simulink model "NDI_and_CA_Model"  (R2012b)
settings: Solver=FixedStepDiscrete  StartTime=0.0  StopTime=inf  FixedStep=T_sim  MaxStep=0.01  RelTol=1e-5
values from neighbouring files (symbols this model uses):
  A_x = 0.015    [SetupComplete.m]
  A_y = A_x    (= 0.015)    [SetupComplete.m]
  A_z = 0.16    [SetupComplete.m]
  C_x = 1.2    [SetupComplete.m]
  C_y = C_x    (= 1.2)    [SetupComplete.m]
  C_z = 2.2    [SetupComplete.m]
  CG_0 = [0,0,0.02]'    [SetupComplete.m]
  eta_23 = deg2rad(-1.42)    [Run3Copter.m]
  g = 9.81    [SetupComplete.m]
  h_M = 0.064    [SetupComplete.m]
  I_BAC_0 = [ Ix,0,Ixz;0,Iy,0;Ixz,0,Iz]    [SetupComplete.m]
  l = 0.345    [SetupComplete.m]
  l_arm = 0.264    [SetupComplete.m]
  m = 3.51    [SetupComplete.m]
  m_0 = 2.61    [SetupComplete.m]
  m_M = 0.300    (= 0.3)    [SetupComplete.m]
  rho = 1.15    [SetupComplete.m]
  Rotation_sign = [ 1,-1,-1]    [SetupComplete.m]
  throtle_1 = 0.512    [Run3Copter.m]
  throtle_23 = throtle_1/cos(eta_23)    [Run3Copter.m]
  Throttle_Hover = X(1)/16    [SetupComplete.m]
libraries: XXCopter_C x24, simulink_extras x21, aerolibutil x3
(part 1 of 2)
settings Model: ExtModeTrigDuration=5000  Creator=DavidTorres  LastModifiedBy=david.torres
settings SolverCC: SolverResetMethod=Robust  PositivePriorityOrder=on
settings DataIOCC: ExternalInput=getinputstruct(op_trim1)  InitialState=getstatestruct(op_trim1)  SignalLoggingSaveFormat=ModelDataLogs  Refine=10
settings OptimizationCC: InlineParams=on  UseFloatMulNetSlope=on  UseSpecifiedMinMax=on  InlineInvariantSignals=on  EnhancedBackFolding=on  PassReuseOutputArgsAs=Individual arguments  RollThreshold=50  ZeroExternalMemoryAtStartup=off  ZeroInternalMemoryAtStartup=off  EfficientMapNaN2IntZero=off  OptimizeModelRefInitCode=on  LifeSpan=1  MaxStackSize=inf  SimCompilerOptimization=On
settings DebuggingCC: SignalInfNanChecking=warning  WriteAfterReadMsg=DisableAll  UnderspecifiedInitializationDetection=Simplified  MergeDetectMultiDrivingBlocksExec=error  CheckMatrixSingularityMsg=warning  IntegerOverflowMsg=error  Int32ToFloatConvMsg=none  ParameterUnderflowMsg=error  ParameterTunabilityLossMsg=error  UnderSpecifiedDataTypeMsg=warning  UniqueDataStoreMsg=error  AssertControl=DisableAll  ModelReferenceIOMsg=error  StrictBusMsg=ErrorOnBusTreatedAsVector  NonBusSignalsTreatedAsBus=error
settings HardwareCC: ProdIntDivRoundTo=Zero  ProdEndianess=LittleEndian  ProdHWDeviceType=Generic->32-bit x86 compatible  TargetBitPerLong=64  TargetBitPerPointer=64  TargetLargestAtomicInteger=Integer  TargetLargestAtomicFloat=Double  TargetIntDivRoundTo=Zero  TargetEndianess=LittleEndian  TargetWordSize=64  TargetHWDeviceType=Intel->x86-64  ProdEqTarget=off
settings RTWCC: SystemTargetFile=ert.tlc  GenCodeOnly=on  TemplateMakefile=RTW.MSVCBuild  Description=Create Visual C/C++ Solution File for the Embedded Coder  GenerateReport=on  ProcessScript=ert_make_rtw_hook  IncludeHyperlinkInReport=on  LaunchReport=on  CodeExecutionProfiling=on  GenerateTraceInfo=on  RTWCompilerOptimization=On  CheckMdlBeforeBuild=Warning
settings CodeAppCC: IgnoreCustomStorageClasses=off  IgnoreTestpoints=on  MATLABSourceComments=on
settings ERTTargetCC: CodeReplacementLibrary=C89/C90 (ANSI)  UtilityFuncGeneration=Shared location  MultiwordLength=2048  GenerateSampleERTMain=on  IncludeMdlTerminateFcn=off  CombineSignalStateStructs=on  SuppressErrorStatus=on  IncludeFileDelimiter=UseQuote  SupportAbsoluteTime=off  MultiInstanceERTCode=on  SupportComplex=off  ParenthesesLevel=Maximum  InlinedParameterPlacement=NonHierarchical  ERTCustomFileTemplate=example_file_process.tlc  GlobalDataDefinition=InSourceFile  DataDefinitionFile=global_vars.c  GlobalDataReference=InSourceFile  PreserveIfCondition=on  SuppressUnreachableDefaultCases=off

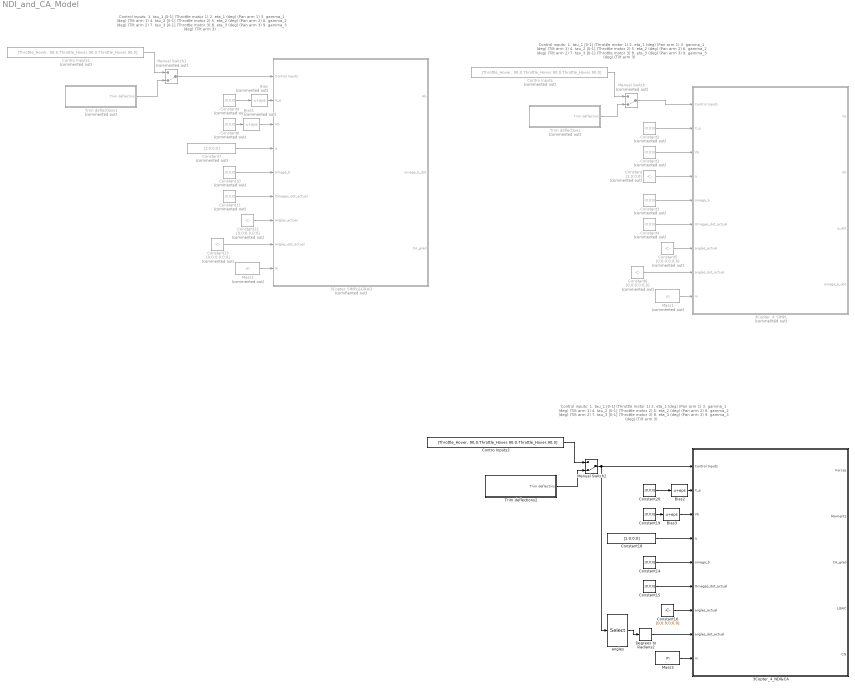
== system NDI_and_CA_Model ==
  note: Control inputs:
      | 1. tau_1 [0-1] (Throttle motor 1)
      | 2. eta_1 (deg)  (Pan arm 1)
      | 3. gamma_1 (deg)  (Tilt arm 1)
      |
      | 4. tau_2 [0-1] (Throttle motor 2)
      | 5. eta_2 (deg)  (Pan arm 2)
      | 6. gamma_2 (deg)  (Tilt arm 2)
      |
      | 7. tau_3 [0-1] (Throttle motor 3)
      | 8. eta_3 (deg)  (Pan arm  3)
      | 9. gamma_3 (deg)  (Tilt arm 3)
  note: Control inputs:
      | 1. tau_1 [0-1] (Throttle motor 1)
      | 2. eta_1 (deg)  (Pan arm 1)
      | 3. gamma_1 (deg)  (Tilt arm 1)
      |
      | 4. tau_2 [0-1] (Throttle motor 2)
      | 5. eta_2 (deg)  (Pan arm 2)
      | 6. gamma_2 (deg)  (Tilt arm 2)
      |
      | 7. tau_3 [0-1] (Throttle motor 3)
      | 8. eta_3 (deg)  (Pan arm  3)
      | 9. gamma_3 (deg)  (Tilt arm 3)
  note: Control inputs:
      | 1. tau_1 [0-1] (Throttle motor 1)
      | 2. eta_1 (deg)  (Pan arm 1)
      | 3. gamma_1 (deg)  (Tilt arm 1)
      |
      | 4. tau_2 [0-1] (Throttle motor 2)
      | 5. eta_2 (deg)  (Pan arm 2)
      | 6. gamma_2 (deg)  (Tilt arm 2)
      |
      | 7. tau_3 [0-1] (Throttle motor 3)
      | 8. eta_3 (deg)  (Pan arm  3)
      | 9. gamma_3 (deg)  (Tilt arm 3)
  3Copter_4_NDI&CA : Subsystem  TreatAsAtomicUnit=on
  3Copter_4_SIMPL : Subsystem  Commented=on  TreatAsAtomicUnit=on
  3Copter_SIMPL&GRAD : Subsystem  Commented=on  TreatAsAtomicUnit=on
  Bias : Bias  Commented=on  Bias=eps
  Bias1 : Bias  Commented=on  Bias=eps
  Bias2 : Bias  Bias=eps
  Bias3 : Bias  Bias=eps
  Constant : Constant  Commented=on  Value=[1;0;0;0]
  Constant{1..4,8..11} (8 alike) : Constant  Commented=on  Value=[0;0;0]
  Constant{5..6,12..13} (4 alike) : Constant  Commented=on  Value=[0;0;0;0;0;0]
  Constant{14..15,19..20} (4 alike) : Constant  Value=[0;0;0]
  Constant16 : Constant  Value=[0;0;0;0;0;0]
  Constant18 : Constant  Value=[1;0;0;0]
  Constant7 : Constant  Commented=on  Value=[1;0;0;0]
  Contro Inputs : Constant  Commented=on  Value=[Throttle_Hover, 90,0,Throttle_Hover,90,0,Throttle_Hover,90,0]
  Contro Inputs1 : Constant  Commented=on  Value=[Throttle_Hover, 90,0,Throttle_Hover,90,0,Throttle_Hover,90,0]
  Contro Inputs2 : Constant  Value=[Throttle_Hover, 90,0,Throttle_Hover,90,0,Throttle_Hover,90,0]
  Degrees to Radians2 : simulink_extras/Transformations/Degrees to Radians
  Manual Switch : ManualSwitch  Commented=on  CurrentSetting=0
  Manual Switch1 : ManualSwitch  Commented=on  CurrentSetting=0
  Manual Switch2 : ManualSwitch  CurrentSetting=0
  Mass1 : Constant  Commented=on  Value=m
  Mass2 : Constant  Commented=on  Value=m
  Mass3 : Constant  Value=m
  Trim deflections : Subsystem  Commented=on  TreatAsAtomicUnit=on
  Trim deflections1 : Subsystem  Commented=on  TreatAsAtomicUnit=on
  Trim deflections2 : Subsystem  TreatAsAtomicUnit=on
  "angles " : Selector  IndexMode=Zero-based  InputPortWidth=9  Indices=[1,2,4,5,7,8]
  wires:
  Manual Switch/1 -> 3Copter_4_SIMPL/1(Control Inputs)
  Contro Inputs/1 -> Manual Switch/1
  Trim deflections/1(Trim deflectins) -> Manual Switch/2
  Constant/1 -> 3Copter_4_SIMPL/4(q)
  Constant1/1 -> 3Copter_4_SIMPL/3(Vb)
  Constant2/1 -> 3Copter_4_SIMPL/2(X_e)
  Constant3/1 -> 3Copter_4_SIMPL/5(omega_b)
  Constant4/1 -> 3Copter_4_SIMPL/6(Omegas_dot_actual)
  Constant5/1 -> 3Copter_4_SIMPL/7(angles_actual)
  Constant6/1 -> 3Copter_4_SIMPL/8(angles_dot_actual)
  Mass1/1 -> 3Copter_4_SIMPL/9(" m")
  Manual Switch1/1 -> 3Copter_SIMPL&GRAD/1(Control Inputs)
  Contro Inputs1/1 -> Manual Switch1/1
  Trim deflections1/1(Trim deflectins) -> Manual Switch1/2
  Constant7/1 -> 3Copter_SIMPL&GRAD/4(q)
  Constant8/1 -> Bias1/1
  Constant9/1 -> Bias/1
  Constant10/1 -> 3Copter_SIMPL&GRAD/5(omega_b)
  Constant11/1 -> 3Copter_SIMPL&GRAD/6(Omegas_dot_actual)
  Constant12/1 -> 3Copter_SIMPL&GRAD/7(angles_actual)
  Constant13/1 -> 3Copter_SIMPL&GRAD/8(angles_dot_actual)
  Mass2/1 -> 3Copter_SIMPL&GRAD/9(" m")
  Bias/1 -> 3Copter_SIMPL&GRAD/2(X_e)
  Bias1/1 -> 3Copter_SIMPL&GRAD/3(Vb)
  Manual Switch2/1 -> 3Copter_4_NDI&CA/1(Control Inputs), "angles "/1
  Contro Inputs2/1 -> Manual Switch2/1
  Trim deflections2/1(Trim deflectins) -> Manual Switch2/2
  Constant18/1 -> 3Copter_4_NDI&CA/4(q)
  Constant19/1 -> Bias3/1
  Constant20/1 -> Bias2/1
  Constant14/1 -> 3Copter_4_NDI&CA/5(omega_b)
  Constant15/1 -> 3Copter_4_NDI&CA/6(Omegas_dot_actual)
  Constant16/1 -> 3Copter_4_NDI&CA/7(angles_actual)
  "angles "/1 -> Degrees to Radians2/1
  Mass3/1 -> 3Copter_4_NDI&CA/9(" m")
  Bias2/1 -> 3Copter_4_NDI&CA/2(X_e)
  Bias3/1 -> 3Copter_4_NDI&CA/3(Vb)
  Degrees to Radians2/1 -> 3Copter_4_NDI&CA/8(angles_dot_actual)

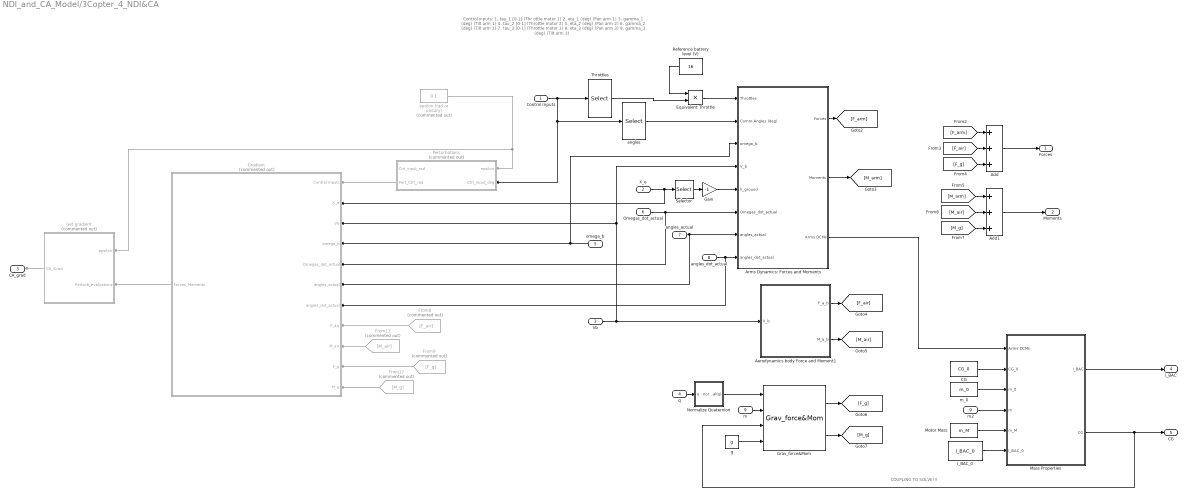
== system NDI_and_CA_Model/3Copter_4_NDI&CA ==
  note: COUPLING TO SOLVE!!!
  note: Control inputs:
      | 1. tau_1 [0-1] (Thr ottle motor 1)
      | 2. eta_1 (deg)  (Pan arm 1)
      | 3. gamma_1 (deg)  (Tilt arm 1)
      |
      | 4. tau_2 [0-1] (Throttle motor 2)
      | 5. eta_2 (deg)  (Pan arm 2)
      | 6. gamma_2 (deg)  (Tilt arm 2)
      |
      | 7. tau_3 [0-1] (Throttle motor 3)
      | 8. eta_3 (deg)  (Pan arm  3)
      | 9. gamma_3 (deg)  (Tilt arm 3)
  Control Inputs : Inport
  X_e : Inport  Port=2
  Vb : Inport  Port=3
  q : Inport  Port=4
  omega_b : Inport  Port=5
  Omegas_dot_actual : Inport  Port=6
  angles_actual : Inport  Port=7
  angles_dot_actual : Inport  Port=8
  " m" : Inport  Port=9
  Add : Sum  Inputs=+++
  Add1 : Sum  Inputs=+++
  Aerodynamics body Force and Moment1 : MATLAB Function  TreatAsAtomicUnit=on
      settings: PermitHierarchicalResolution=ParametersOnly
  Arms Dynamics: Forces and Moments : Subsystem  TreatAsAtomicUnit=on
  CG : Constant  Value=CG_0
  Equivalent Throttle : Product  Inputs=**
  From11 : From  Commented=on  GotoTag=M_air
  From12 : From  Commented=on  GotoTag=M_g
  From8 : From  Commented=on  GotoTag=F_air
  From9 : From  Commented=on  GotoTag=F_g
  Gain : Gain  Gain=-1
  Get gradient : MATLAB Function  Commented=on  TreatAsAtomicUnit=on
      settings: PermitHierarchicalResolution=ParametersOnly
  Gradient : Subsystem  Commented=on  TreatAsAtomicUnit=on
  Grav_force&Mom : XXCopter_C/Grav_force&Mom
  I_BAC_0 : Constant  Value=I_BAC_0
  Mass Properties : Subsystem  TreatAsAtomicUnit=on
  Motor Mass : Constant  Value=m_M
  Normalize Quaternion : Subsystem  TreatAsAtomicUnit=on
  Perturbations : MATLAB Function  Commented=on  TreatAsAtomicUnit=on
      settings: PermitHierarchicalResolution=ParametersOnly
  Reference batrery level (V) : Constant  Value=16
  Selector : Selector  IndexMode=Zero-based  InputPortWidth=3  Indices=2
  Throttles : Selector  IndexMode=Zero-based  InputPortWidth=9  Indices=[0,3,6]
  "angles " : Selector  IndexMode=Zero-based  InputPortWidth=9  Indices=[1,2,4,5,7,8]
  epsilon (rad or unitary) : Constant  Commented=on  Value=0.1
  g : Constant  Value=g
  m2 : InportShadow  Port=9
  m_0 : Constant  Value=m_0
  Forces : Outport
  Moments : Outport  Port=2
  CA_grad : Outport  Port=3
  I_BAC : Outport  Port=4
  "CG " : Outport  Port=5
  wires:
  Vb/1 -> Arms Dynamics: Forces and Moments/4(V_b), Gradient/3(Vb), Aerodynamics body Force and Moment1/1(V_b)
  omega_b/1 -> Arms Dynamics: Forces and Moments/3(omega_b), Gradient/4(omega_b)
  " m"/1 -> Grav_force&Mom/2
  X_e/1 -> Gradient/2(X_e), Selector/1
  Selector/1 -> Gain/1
  Gain/1 -> Arms Dynamics: Forces and Moments/5(h_ground)
  Arms Dynamics: Forces and Moments/1(Forces) -> [F_arm]
  Arms Dynamics: Forces and Moments/2(Moments) -> [M_arm]
  Aerodynamics body Force and Moment1/1(F_a_b) -> [F_air]
  Aerodynamics body Force and Moment1/2(M_a_b) -> [M_air]
  Grav_force&Mom/1 -> [F_g]
  Grav_force&Mom/2 -> [M_g]
  [F_arm] -> Add/1
  [F_air] -> Add/2
  [F_g] -> Add/3
  [M_arm] -> Add1/1
  [M_g] -> Add1/3
  [M_air] -> Add1/2
  Throttles/1 -> Equivalent Throttle/2
  Control Inputs/1 -> Throttles/1, "angles "/1, Perturbations/2(Ctrl_input_deg)
  "angles "/1 -> Arms Dynamics: Forces and Moments/2(Comm Angles (deg))
  Arms Dynamics: Forces and Moments/3(Arms DCMs) -> Mass Properties/1(Arms DCMs)
  CG/1 -> Mass Properties/2(CG_0)
  Motor Mass/1 -> Mass Properties/5(m_M)
  I_BAC_0/1 -> Mass Properties/6(I_BAC_0)
  m_0/1 -> Mass Properties/3(m_0)
  m2/1 -> Mass Properties/4(m)
  Add/1 -> Forces/1
  Mass Properties/2(CG) -> "CG "/1, Grav_force&Mom/3
  Equivalent Throttle/1 -> Arms Dynamics: Forces and Moments/1(Throttles)
  Reference batrery level (V)/1 -> Equivalent Throttle/1
  Add1/1 -> Moments/1
  q/1 -> Normalize Quaternion/1(q)
  Omegas_dot_actual/1 -> Gradient/5(Omegas_dot_actual), Arms Dynamics: Forces and Moments/6(Omegas_dot_actual)
  angles_dot_actual/1 -> Gradient/7(angles_dot_actual), Arms Dynamics: Forces and Moments/8(angles_dot_actual)
  angles_actual/1 -> Gradient/6(angles_actual), Arms Dynamics: Forces and Moments/7(angles_actual)
  g/1 -> Grav_force&Mom/4
  Normalize Quaternion/1(normal(q)) -> Grav_force&Mom/1
  From12/1 -> Gradient/11(M_g)
  From11/1 -> Gradient/9(M_air)
  From8/1 -> Gradient/8(F_air)
  From9/1 -> Gradient/10(F_g)
  Mass Properties/1(I_BAC) -> I_BAC/1
  Gradient/1(Forces_Moments) -> Get gradient/2(Perturb_evaluations)
  Perturbations/2(Pert_Ctrl_rad) -> Gradient/1("Control Inputs ")
  epsilon (rad or unitary)/1 -> Get gradient/1(epsilon), Perturbations/1(epsilon)
  Get gradient/1(CA_Grad) -> CA_grad/1

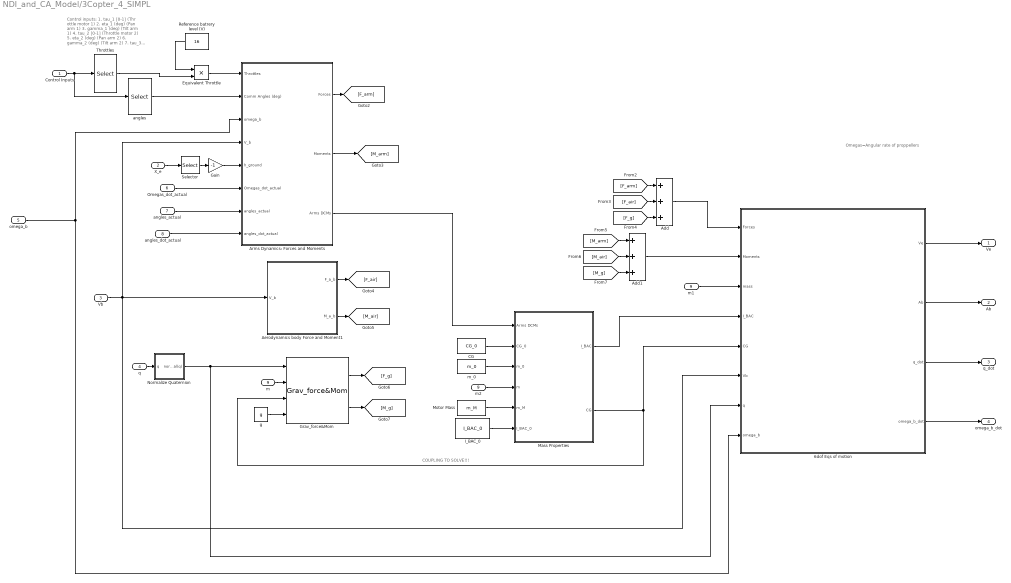
== system NDI_and_CA_Model/3Copter_4_SIMPL ==
  note: COUPLING TO SOLVE!!!
  note: Omegas=Angular rate of proppellers
  note: Control inputs:
      | 1. tau_1 [0-1] (Thr ottle motor 1)
      | 2. eta_1 (deg)  (Pan arm 1)
      | 3. gamma_1 (deg)  (Tilt arm 1)
      |
      | 4. tau_2 [0-1] (Throttle motor 2)
      | 5. eta_2 (deg)  (Pan arm 2)
      | 6. gamma_2 (deg)  (Tilt arm 2)
      |
      | 7. tau_3 [0-1] (Throttle motor 3)
      | 8. eta_3 (deg)  (Pan arm  3)
      | 9. gamma_3 (deg)  (Tilt arm 3)
  Control Inputs : Inport
  X_e : Inport  Port=2
  Vb : Inport  Port=3
  q : Inport  Port=4
  omega_b : Inport  Port=5
  Omegas_dot_actual : Inport  Port=6
  angles_actual : Inport  Port=7
  angles_dot_actual : Inport  Port=8
  " m" : Inport  Port=9
  6dof Eqs of motion : Subsystem  TreatAsAtomicUnit=on
  Add : Sum  Inputs=+++
  Add1 : Sum  Inputs=+++
  Aerodynamics body Force and Moment1 : MATLAB Function  TreatAsAtomicUnit=on
      settings: PermitHierarchicalResolution=ParametersOnly
  Arms Dynamics: Forces and Moments : Subsystem  TreatAsAtomicUnit=on
  CG : Constant  Value=CG_0
  Equivalent Throttle : Product  Inputs=**
  Gain : Gain  Gain=-1
  Grav_force&Mom : XXCopter_C/Grav_force&Mom
  I_BAC_0 : Constant  Value=I_BAC_0
  Mass Properties : Subsystem  TreatAsAtomicUnit=on
  Motor Mass : Constant  Value=m_M
  Normalize Quaternion : Subsystem  TreatAsAtomicUnit=on
  Reference batrery level (V) : Constant  Value=16
  Selector : Selector  IndexMode=Zero-based  InputPortWidth=3  Indices=2
  Throttles : Selector  IndexMode=Zero-based  InputPortWidth=9  Indices=[0,3,6]
  "angles " : Selector  IndexMode=Zero-based  InputPortWidth=9  Indices=[1,2,4,5,7,8]
  g : Constant  Value=g
  m1 : InportShadow  Port=9
  m2 : InportShadow  Port=9
  m_0 : Constant  Value=m_0
  Ve : Outport
  Ab : Outport  Port=2
  q_dot : Outport  Port=3
  omega_b_dot : Outport  Port=4
  wires:
  m1/1 -> 6dof Eqs of motion/3(mass)
  Vb/1 -> Arms Dynamics: Forces and Moments/4(V_b), Aerodynamics body Force and Moment1/1(V_b), 6dof Eqs of motion/6(Vb)
  omega_b/1 -> Arms Dynamics: Forces and Moments/3(omega_b), 6dof Eqs of motion/8(omega_b)
  " m"/1 -> Grav_force&Mom/2
  X_e/1 -> Selector/1
  Selector/1 -> Gain/1
  Gain/1 -> Arms Dynamics: Forces and Moments/5(h_ground)
  Arms Dynamics: Forces and Moments/1(Forces) -> [F_arm]
  Arms Dynamics: Forces and Moments/2(Moments) -> [M_arm]
  Aerodynamics body Force and Moment1/1(F_a_b) -> [F_air]
  Aerodynamics body Force and Moment1/2(M_a_b) -> [M_air]
  Grav_force&Mom/1 -> [F_g]
  Grav_force&Mom/2 -> [M_g]
  [F_arm] -> Add/1
  [F_air] -> Add/2
  [F_g] -> Add/3
  [M_arm] -> Add1/1
  [M_g] -> Add1/3
  [M_air] -> Add1/2
  Throttles/1 -> Equivalent Throttle/2
  Control Inputs/1 -> Throttles/1, "angles "/1
  "angles "/1 -> Arms Dynamics: Forces and Moments/2(Comm Angles (deg))
  Arms Dynamics: Forces and Moments/3(Arms DCMs) -> Mass Properties/1(Arms DCMs)
  CG/1 -> Mass Properties/2(CG_0)
  Motor Mass/1 -> Mass Properties/5(m_M)
  I_BAC_0/1 -> Mass Properties/6(I_BAC_0)
  m_0/1 -> Mass Properties/3(m_0)
  m2/1 -> Mass Properties/4(m)
  Add/1 -> 6dof Eqs of motion/1(Forces)
  Mass Properties/2(CG) -> Grav_force&Mom/3, 6dof Eqs of motion/5(CG)
  Mass Properties/1(I_BAC) -> 6dof Eqs of motion/4(I_BAC)
  Equivalent Throttle/1 -> Arms Dynamics: Forces and Moments/1(Throttles)
  Reference batrery level (V)/1 -> Equivalent Throttle/1
  Add1/1 -> 6dof Eqs of motion/2(Moments)
  6dof Eqs of motion/1(Ve) -> Ve/1
  6dof Eqs of motion/2(Ab) -> Ab/1
  6dof Eqs of motion/3("q_dot ") -> q_dot/1
  6dof Eqs of motion/4(omega_b_dot) -> omega_b_dot/1
  q/1 -> Normalize Quaternion/1(q)
  Omegas_dot_actual/1 -> Arms Dynamics: Forces and Moments/6(Omegas_dot_actual)
  angles_dot_actual/1 -> Arms Dynamics: Forces and Moments/8(angles_dot_actual)
  angles_actual/1 -> Arms Dynamics: Forces and Moments/7(angles_actual)
  g/1 -> Grav_force&Mom/4
  Normalize Quaternion/1(normal(q)) -> Grav_force&Mom/1, 6dof Eqs of motion/7(q)

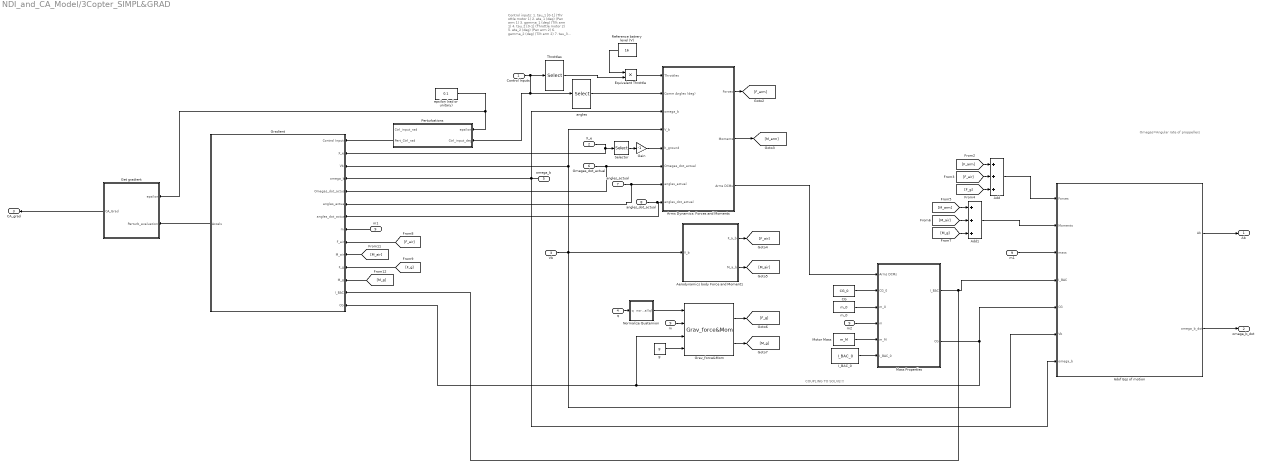
== system NDI_and_CA_Model/3Copter_SIMPL&GRAD ==
  note: COUPLING TO SOLVE!!!
  note: Omegas=Angular rate of proppellers
  note: Control inputs:
      | 1. tau_1 [0-1] (Thr ottle motor 1)
      | 2. eta_1 (deg)  (Pan arm 1)
      | 3. gamma_1 (deg)  (Tilt arm 1)
      |
      | 4. tau_2 [0-1] (Throttle motor 2)
      | 5. eta_2 (deg)  (Pan arm 2)
      | 6. gamma_2 (deg)  (Tilt arm 2)
      |
      | 7. tau_3 [0-1] (Throttle motor 3)
      | 8. eta_3 (deg)  (Pan arm  3)
      | 9. gamma_3 (deg)  (Tilt arm 3)
  Control Inputs : Inport
  X_e : Inport  Port=2
  Vb : Inport  Port=3
  q : Inport  Port=4
  omega_b : Inport  Port=5
  Omegas_dot_actual : Inport  Port=6
  angles_actual : Inport  Port=7
  angles_dot_actual : Inport  Port=8
  " m" : Inport  Port=9
  " m1" : InportShadow  Port=9
  6dof Eqs of motion : Subsystem  TreatAsAtomicUnit=on
  Add : Sum  Inputs=+++
  Add1 : Sum  Inputs=+++
  Aerodynamics body Force and Moment1 : MATLAB Function  TreatAsAtomicUnit=on
      settings: PermitHierarchicalResolution=ParametersOnly
  Arms Dynamics: Forces and Moments : Subsystem  TreatAsAtomicUnit=on
  CG : Constant  Value=CG_0
  Equivalent Throttle : Product  Inputs=**
  Gain : Gain  Gain=-1
  Get gradient : MATLAB Function  TreatAsAtomicUnit=on
      settings: PermitHierarchicalResolution=ParametersOnly
  Gradient : Subsystem  TreatAsAtomicUnit=on
  Grav_force&Mom : XXCopter_C/Grav_force&Mom
  I_BAC_0 : Constant  Value=I_BAC_0
  Mass Properties : Subsystem  TreatAsAtomicUnit=on
  Motor Mass : Constant  Value=m_M
  Normalize Quaternion : Subsystem  TreatAsAtomicUnit=on
  Perturbations : MATLAB Function  TreatAsAtomicUnit=on
      settings: PermitHierarchicalResolution=ParametersOnly
  Reference batrery level (V) : Constant  Value=16
  Selector : Selector  IndexMode=Zero-based  InputPortWidth=3  Indices=2
  Throttles : Selector  IndexMode=Zero-based  InputPortWidth=9  Indices=[0,3,6]
  "angles " : Selector  IndexMode=Zero-based  InputPortWidth=9  Indices=[1,2,4,5,7,8]
  epsilon (rad or unitary) : Constant  Value=0.1
  g : Constant  Value=g
  m1 : InportShadow  Port=9
  m2 : InportShadow  Port=9
  m_0 : Constant  Value=m_0
  Ab : Outport
  omega_b_dot : Outport  Port=2
  CA_grad : Outport  Port=3
  wires:
  m1/1 -> 6dof Eqs of motion/3(mass)
  Vb/1 -> Arms Dynamics: Forces and Moments/4(V_b), Gradient/3(Vb), Aerodynamics body Force and Moment1/1(V_b), 6dof Eqs of motion/6(Vb)
  omega_b/1 -> 6dof Eqs of motion/7(omega_b), Gradient/4(omega_b), Arms Dynamics: Forces and Moments/3(omega_b)
  " m"/1 -> Grav_force&Mom/2
  X_e/1 -> Gradient/2(X_e), Selector/1
  Selector/1 -> Gain/1
  Gain/1 -> Arms Dynamics: Forces and Moments/5(h_ground)
  Arms Dynamics: Forces and Moments/1(Forces) -> [F_arm]
  Arms Dynamics: Forces and Moments/2(Moments) -> [M_arm]
  Aerodynamics body Force and Moment1/1(F_a_b) -> [F_air]
  Aerodynamics body Force and Moment1/2(M_a_b) -> [M_air]
  Grav_force&Mom/1 -> [F_g]
  Grav_force&Mom/2 -> [M_g]
  [F_arm] -> Add/1
  [F_air] -> Add/2
  [F_g] -> Add/3
  [M_arm] -> Add1/1
  [M_g] -> Add1/3
  [M_air] -> Add1/2
  Throttles/1 -> Equivalent Throttle/2
  Control Inputs/1 -> Throttles/1, Perturbations/2(Ctrl_input_deg), "angles "/1
  "angles "/1 -> Arms Dynamics: Forces and Moments/2(Comm Angles (deg))
  Arms Dynamics: Forces and Moments/3(Arms DCMs) -> Mass Properties/1(Arms DCMs)
  CG/1 -> Mass Properties/2(CG_0)
  Motor Mass/1 -> Mass Properties/5(m_M)
  I_BAC_0/1 -> Mass Properties/6(I_BAC_0)
  m_0/1 -> Mass Properties/3(m_0)
  m2/1 -> Mass Properties/4(m)
  Add/1 -> 6dof Eqs of motion/1(Forces)
  Mass Properties/2(CG) -> Gradient/14(CG), Grav_force&Mom/3, 6dof Eqs of motion/5(CG)
  Equivalent Throttle/1 -> Arms Dynamics: Forces and Moments/1(Throttles)
  Reference batrery level (V)/1 -> Equivalent Throttle/1
  Add1/1 -> 6dof Eqs of motion/2(Moments)
  6dof Eqs of motion/2(omega_b_dot) -> omega_b_dot/1
  q/1 -> Normalize Quaternion/1(q)
  Omegas_dot_actual/1 -> Arms Dynamics: Forces and Moments/6(Omegas_dot_actual), Gradient/5(Omegas_dot_actual)
  angles_dot_actual/1 -> Gradient/7(angles_dot_actual), Arms Dynamics: Forces and Moments/8(angles_dot_actual)
  angles_actual/1 -> Arms Dynamics: Forces and Moments/7(angles_actual), Gradient/6(angles_actual)
  g/1 -> Grav_force&Mom/4
  Normalize Quaternion/1(normal(q)) -> Grav_force&Mom/1
  6dof Eqs of motion/1(Ab) -> Ab/1
  " m1"/1 -> Gradient/8(" m")
  [M_g] -> Gradient/12(M_g)
  [M_air] -> Gradient/10(M_air)
  [F_air] -> Gradient/9(F_air)
  [F_g] -> Gradient/11(F_g)
  Mass Properties/1(I_BAC) -> Gradient/13(I_BAC), 6dof Eqs of motion/4(I_BAC)
  Gradient/1(Accels) -> Get gradient/2(Perturb_evaluations)
  Perturbations/2(Pert_Ctrl_rad) -> Gradient/1("Control Inputs ")
  epsilon (rad or unitary)/1 -> Get gradient/1(epsilon), Perturbations/1(epsilon)
  Get gradient/1(CA_Grad) -> CA_grad/1

== system NDI_and_CA_Model/Trim deflections ==
  " " : simulink_extras/Transformations/Radians to Degrees
  Contro Inputs1 : Constant  Value=throtle_1
  Contro Inputs2 : Constant  Value=throtle_23
  Contro Inputs3 : Constant  Value=eta_23
  Gain : Gain  Gain=-1
  Ground : Ground
  Mux : Mux  Inputs=9
  Trim deflectins : Outport
  wires:
  Contro Inputs1/1 -> Mux/1
  Contro Inputs2/1 -> Mux/7, Mux/4
  Ground/1 -> Mux/2, Mux/6, Mux/9, Mux/3
  Contro Inputs3/1 -> " "/1
  " "/1 -> Gain/1, Mux/5
  Gain/1 -> Mux/8
  Mux/1 -> Trim deflectins/1

== system NDI_and_CA_Model/Trim deflections1 ==
  " " : simulink_extras/Transformations/Radians to Degrees
  Contro Inputs1 : Constant  Value=throtle_1
  Contro Inputs2 : Constant  Value=throtle_23
  Contro Inputs3 : Constant  Value=eta_23
  Gain : Gain  Gain=-1
  Ground : Ground
  Mux : Mux  Inputs=9
  Trim deflectins : Outport
  wires:
  Contro Inputs1/1 -> Mux/1
  Contro Inputs2/1 -> Mux/7, Mux/4
  Ground/1 -> Mux/2, Mux/6, Mux/9, Mux/3
  Contro Inputs3/1 -> " "/1
  " "/1 -> Gain/1, Mux/5
  Gain/1 -> Mux/8
  Mux/1 -> Trim deflectins/1

== system NDI_and_CA_Model/Trim deflections2 ==
  " " : simulink_extras/Transformations/Radians to Degrees
  Contro Inputs1 : Constant  Value=throtle_1
  Contro Inputs2 : Constant  Value=throtle_23
  Contro Inputs3 : Constant  Value=eta_23
  Gain : Gain  Gain=-1
  Ground : Ground
  Mux : Mux  Inputs=9
  Trim deflectins : Outport
  wires:
  Contro Inputs1/1 -> Mux/1
  Contro Inputs2/1 -> Mux/7, Mux/4
  Ground/1 -> Mux/2, Mux/6, Mux/9, Mux/3
  Contro Inputs3/1 -> " "/1
  " "/1 -> Gain/1, Mux/5
  Gain/1 -> Mux/8
  Mux/1 -> Trim deflectins/1

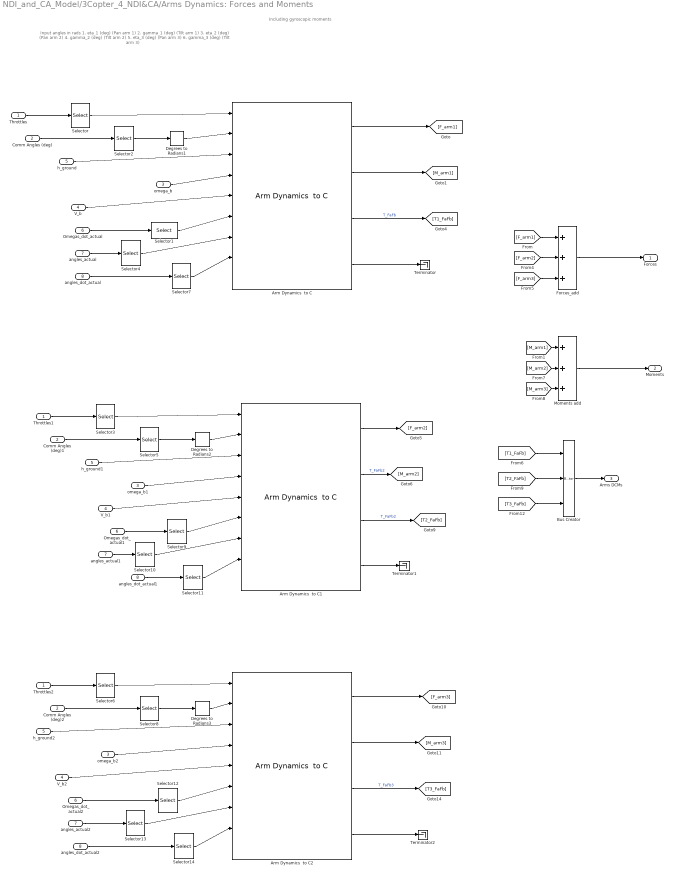
== system NDI_and_CA_Model/3Copter_4_NDI&CA/Arms Dynamics: Forces and Moments ==
  note: Including gyroscopic moments
  note: Input angles in rads
      |
      | 1. eta_1 (deg)  (Pan arm 1)
      | 2. gamma_1 (deg)  (Tilt arm 1)
      |
      | 3. eta_2 (deg)  (Pan arm 2)
      | 4. gamma_2 (deg)  (Tilt arm 2)
      |
      | 5. eta_3 (deg)  (Pan arm  3)
      | 6. gamma_3 (deg)  (Tilt arm 3)
  Throttles : Inport
  Comm Angles (deg) : Inport  Port=2
  omega_b : Inport  Port=3
  V_b : Inport  Port=4
  h_ground : Inport  Port=5
  Omegas_dot_actual : Inport  Port=6
  angles_actual : Inport  Port=7
  angles_dot_actual : Inport  Port=8
  Arm Dynamics  to C : XXCopter_C/Arm Dynamics  to C  Rot_sign=Rotation_sign(1)  arm_hub_pos=l*[1;0;0]  Arm_axis=[l_arm;0;0]  arm_num=1  eta_dir=[1;0;0]  gamma_dir=[0;1;0]  J_T=J_T  J_FA=J_FA  h=h  switch_val=direct_feedforward  omega_n=35  xi=1.45  eta_inf_lim=deg2rad(-180)  eta_sup_lim=deg2rad(180)  gamma_inf_lim=deg2rad(-90)  gamma_sup_lim=deg2rad(30)
      link override ESC+Motor Dynamcis  to C/2-D Torque-Throttle-Omega Map: BreakpointsForDimension1=Torque_TTO_vec  BreakpointsForDimension2=Throtle_TTO_vec
  Arm Dynamics  to C1 : XXCopter_C/Arm Dynamics  to C  Rot_sign=Rotation_sign(2)  arm_hub_pos=l*[-1/2;sqrt(3)/2;0]  Arm_axis=[0;l_arm;0]  arm_num=2  eta_dir=[0;1;0]  gamma_dir=[1;0;0]  J_T=J_T  J_FA=J_FA  h=h  switch_val=direct_feedforward  omega_n=35  xi=1.45  eta_inf_lim=deg2rad(-180)  eta_sup_lim=deg2rad(180)  gamma_inf_lim=deg2rad(-30)  gamma_sup_lim=deg2rad(90)
  Arm Dynamics  to C2 : XXCopter_C/Arm Dynamics  to C  Rot_sign=Rotation_sign(3)  arm_hub_pos=l*[-1/2;-sqrt(3)/2;0]  Arm_axis=[0;-l_arm;0]  arm_num=3  eta_dir=[0;1;0]  gamma_dir=[1;0;0]  J_T=J_T  J_FA=J_FA  h=h  switch_val=direct_feedforward  omega_n=35  xi=1.45  eta_inf_lim=deg2rad(-180)  eta_sup_lim=deg2rad(180)  gamma_inf_lim=deg2rad(-90)  gamma_sup_lim=deg2rad(30)
  Bus Creator : BusCreator  Inputs=3
  Comm Angles (deg)1 : InportShadow  Port=2
  Comm Angles (deg)2 : InportShadow  Port=2
  Degrees to Radians1 : simulink_extras/Transformations/Degrees to Radians
  Degrees to Radians2 : simulink_extras/Transformations/Degrees to Radians
  Degrees to Radians3 : simulink_extras/Transformations/Degrees to Radians
  Forces_add : Sum  Inputs=+++
  Moments add : Sum  Inputs=+++
  Omegas_dot_actual1 : InportShadow  Port=6
  Omegas_dot_actual2 : InportShadow  Port=6
  Selector : Selector  IndexMode=Zero-based  InputPortWidth=3  Indices=0
  Selector1 : Selector  IndexMode=Zero-based  InputPortWidth=3  Indices=0
  Selector10 : Selector  IndexMode=Zero-based  InputPortWidth=6  Indices=[2,3]
  Selector11 : Selector  IndexMode=Zero-based  InputPortWidth=6  Indices=[2,3]
  Selector12 : Selector  IndexMode=Zero-based  InputPortWidth=3  Indices=2
  Selector13 : Selector  IndexMode=Zero-based  InputPortWidth=6  Indices=[4,5]
  Selector14 : Selector  IndexMode=Zero-based  InputPortWidth=6  Indices=[4,5]
  Selector2 : Selector  IndexMode=Zero-based  InputPortWidth=6  Indices=[0,1]
  Selector3 : Selector  IndexMode=Zero-based  InputPortWidth=3
  Selector4 : Selector  IndexMode=Zero-based  InputPortWidth=6  Indices=[0,1]
  Selector5 : Selector  IndexMode=Zero-based  InputPortWidth=6  Indices=[2,3]
  Selector6 : Selector  IndexMode=Zero-based  InputPortWidth=3  Indices=2
  Selector7 : Selector  IndexMode=Zero-based  InputPortWidth=6  Indices=[0,1]
  Selector8 : Selector  IndexMode=Zero-based  InputPortWidth=6  Indices=[4,5]
  Selector9 : Selector  IndexMode=Zero-based  InputPortWidth=3
  Terminator : Terminator
  Terminator1 : Terminator
  Terminator2 : Terminator
  Throttles1 : InportShadow
  Throttles2 : InportShadow
  V_b1 : InportShadow  Port=4
  V_b2 : InportShadow  Port=4
  angles_actual1 : InportShadow  Port=7
  angles_actual2 : InportShadow  Port=7
  angles_dot_actual1 : InportShadow  Port=8
  angles_dot_actual2 : InportShadow  Port=8
  h_ground1 : InportShadow  Port=5
  h_ground2 : InportShadow  Port=5
  omega_b1 : InportShadow  Port=3
  omega_b2 : InportShadow  Port=3
  Forces : Outport
  Moments : Outport  Port=2
  Arms DCMs : Outport  Port=3
  wires:
  Throttles/1 -> Selector/1
  Selector/1 -> Arm Dynamics  to C/1
  V_b/1 -> Arm Dynamics  to C/5
  Forces_add/1 -> Forces/1
  Moments add/1 -> Moments/1
  h_ground/1 -> Arm Dynamics  to C/3
  Arm Dynamics  to C/1 -> [F_arm1]
  Arm Dynamics  to C/2 -> [M_arm1]
  [F_arm1] -> Forces_add/1
  [M_arm1] -> Moments add/1
  omega_b/1 -> Arm Dynamics  to C/4
  [F_arm2] -> Forces_add/2
  [F_arm3] -> Forces_add/3
  [M_arm3] -> Moments add/3
  [M_arm2] -> Moments add/2
  Degrees to Radians1/1 -> Arm Dynamics  to C/2
  Comm Angles (deg)/1 -> Selector2/1
  Selector2/1 -> Degrees to Radians1/1
  Arm Dynamics  to C/3 -> [T1_FaFb]  "T_FaFb"
  Throttles1/1 -> Selector3/1
  Selector3/1 -> Arm Dynamics  to C1/1
  V_b1/1 -> Arm Dynamics  to C1/5
  h_ground1/1 -> Arm Dynamics  to C1/3
  omega_b1/1 -> Arm Dynamics  to C1/4
  Degrees to Radians2/1 -> Arm Dynamics  to C1/2
  Comm Angles (deg)1/1 -> Selector5/1
  Selector5/1 -> Degrees to Radians2/1
  Arm Dynamics  to C1/3 -> [T2_FaFb]  "T_FaFb2"
  Throttles2/1 -> Selector6/1
  Selector6/1 -> Arm Dynamics  to C2/1
  V_b2/1 -> Arm Dynamics  to C2/5
  h_ground2/1 -> Arm Dynamics  to C2/3
  Arm Dynamics  to C2/1 -> [F_arm3]
  Arm Dynamics  to C2/2 -> [M_arm3]
  omega_b2/1 -> Arm Dynamics  to C2/4
  Degrees to Radians3/1 -> Arm Dynamics  to C2/2
  Comm Angles (deg)2/1 -> Selector8/1
  Selector8/1 -> Degrees to Radians3/1
  Arm Dynamics  to C2/3 -> [T3_FaFb]  "T_FaFb3"
  Arm Dynamics  to C/4 -> Terminator/1
  Arm Dynamics  to C1/4 -> Terminator1/1
  Arm Dynamics  to C2/4 -> Terminator2/1
  Arm Dynamics  to C1/1 -> [F_arm2]
  Arm Dynamics  to C1/2 -> [M_arm2]  "T_FaFb2"
  Bus Creator/1 -> Arms DCMs/1
  [T1_FaFb] -> Bus Creator/1
  [T2_FaFb] -> Bus Creator/2
  [T3_FaFb] -> Bus Creator/3
  Omegas_dot_actual/1 -> Selector1/1
  Selector1/1 -> Arm Dynamics  to C/6
  angles_actual/1 -> Selector4/1
  Selector4/1 -> Arm Dynamics  to C/7
  angles_dot_actual/1 -> Selector7/1
  Selector7/1 -> Arm Dynamics  to C/8
  Omegas_dot_actual1/1 -> Selector9/1
  Selector9/1 -> Arm Dynamics  to C1/6
  Selector10/1 -> Arm Dynamics  to C1/7
  angles_dot_actual1/1 -> Selector11/1
  angles_actual1/1 -> Selector10/1
  Selector11/1 -> Arm Dynamics  to C1/8
  Omegas_dot_actual2/1 -> Selector12/1
  Selector12/1 -> Arm Dynamics  to C2/6
  Selector13/1 -> Arm Dynamics  to C2/7
  angles_dot_actual2/1 -> Selector14/1
  angles_actual2/1 -> Selector13/1
  Selector14/1 -> Arm Dynamics  to C2/8

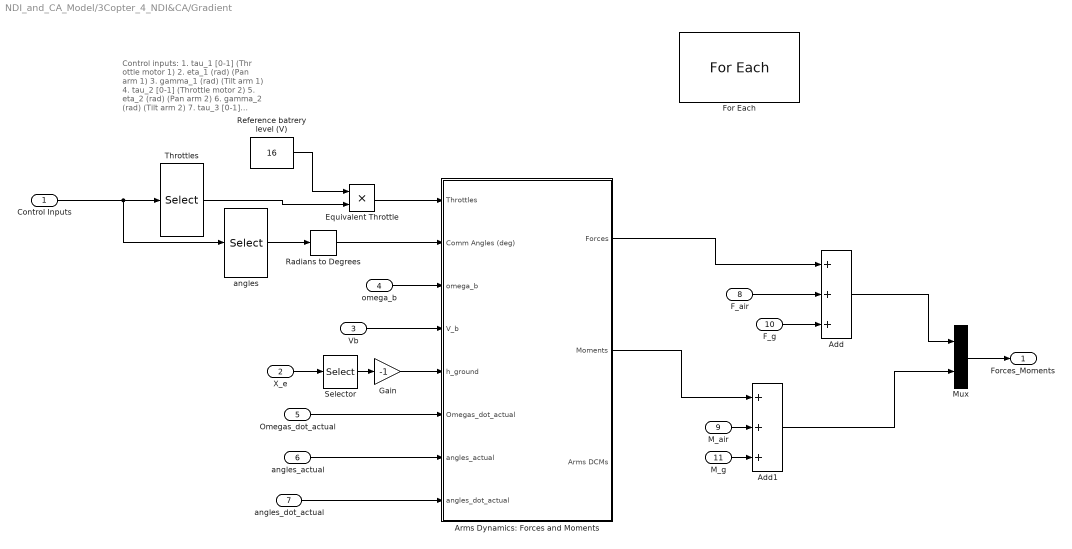
== system NDI_and_CA_Model/3Copter_4_NDI&CA/Gradient ==
  note: Control inputs:
      | 1. tau_1 [0-1] (Thr ottle motor 1)
      | 2. eta_1 (rad)  (Pan arm 1)
      | 3. gamma_1 (rad)  (Tilt arm 1)
      |
      | 4. tau_2 [0-1] (Throttle motor 2)
      | 5. eta_2 (rad)  (Pan arm 2)
      | 6. gamma_2 (rad)  (Tilt arm 2)
      |
      | 7. tau_3 [0-1] (Throttle motor 3)
      | 8. eta_3 (rad)  (Pan arm  3)
      | 9. gamma_3 (rad)  (Tilt arm 3)
  "Control Inputs " : Inport  Partition=on  PartitionDimension=1  PartitionWidth=9
  X_e : Inport  Port=2  Partition=off
  Vb : Inport  Port=3  Partition=off
  omega_b : Inport  Port=4  Partition=off
  Omegas_dot_actual : Inport  Port=5  Partition=off
  angles_actual : Inport  Port=6  Partition=off
  angles_dot_actual : Inport  Port=7  Partition=off
  F_air : Inport  Port=8  Partition=off
  M_air : Inport  Port=9  Partition=off
  F_g : Inport  Port=10  Partition=off
  M_g : Inport  Port=11  Partition=off
  Add : Sum  Inputs=+++
  Add1 : Sum  Inputs=+++
  Arms Dynamics: Forces and Moments : Subsystem  TreatAsAtomicUnit=on
  Equivalent Throttle : Product  Inputs=**
  For Each : ForEach  DisableCoverage=on  IndexMode=One-based
  Gain : Gain  Gain=-1
  Mux : Mux  Inputs=[3,3]
  Radians to Degrees : simulink_extras/Transformations/Radians to Degrees
  Reference batrery level (V) : Constant  Value=16
  Selector : Selector  IndexMode=Zero-based  InputPortWidth=3  Indices=2
  Throttles : Selector  IndexMode=Zero-based  InputPortWidth=9  Indices=[0,3,6]
  "angles " : Selector  IndexMode=Zero-based  InputPortWidth=9  Indices=[1,2,4,5,7,8]
  Forces_Moments : Outport  ConcatenationDimension=2
  wires:
  Vb/1 -> Arms Dynamics: Forces and Moments/4(V_b)
  omega_b/1 -> Arms Dynamics: Forces and Moments/3(omega_b)
  X_e/1 -> Selector/1
  Selector/1 -> Gain/1
  Gain/1 -> Arms Dynamics: Forces and Moments/5(h_ground)
  F_air/1 -> Add/2
  Arms Dynamics: Forces and Moments/1(Forces) -> Add/1
  F_g/1 -> Add/3
  Arms Dynamics: Forces and Moments/2(Moments) -> Add1/1
  M_g/1 -> Add1/3
  M_air/1 -> Add1/2
  Throttles/1 -> Equivalent Throttle/2
  "Control Inputs "/1 -> Throttles/1, "angles "/1
  "angles "/1 -> Radians to Degrees/1
  Add/1 -> Mux/1
  Equivalent Throttle/1 -> Arms Dynamics: Forces and Moments/1(Throttles)
  Reference batrery level (V)/1 -> Equivalent Throttle/1
  Add1/1 -> Mux/2
  Omegas_dot_actual/1 -> Arms Dynamics: Forces and Moments/6(Omegas_dot_actual)
  angles_dot_actual/1 -> Arms Dynamics: Forces and Moments/8(angles_dot_actual)
  angles_actual/1 -> Arms Dynamics: Forces and Moments/7(angles_actual)
  Mux/1 -> Forces_Moments/1
  Radians to Degrees/1 -> Arms Dynamics: Forces and Moments/2(Comm Angles (deg))

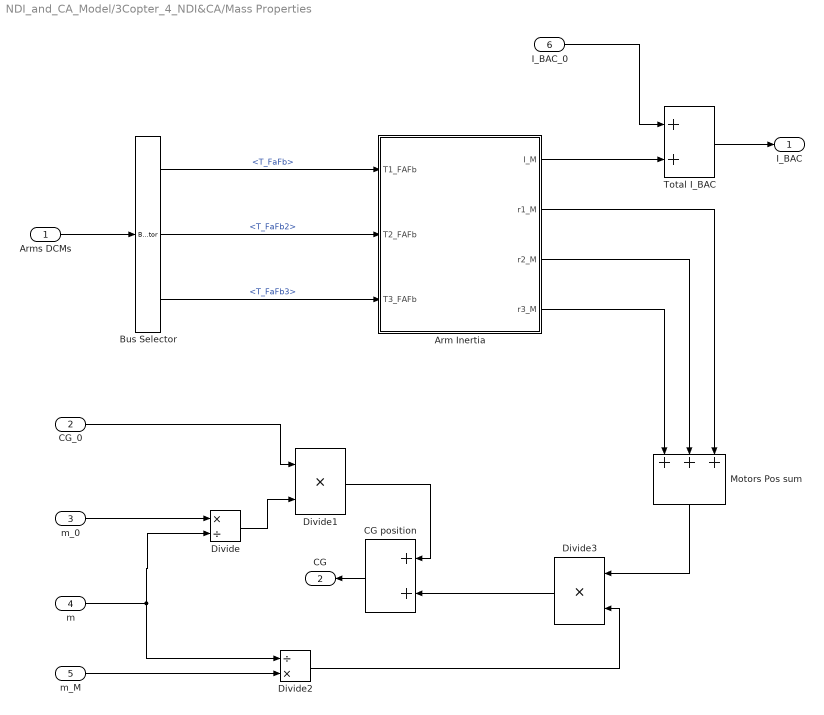
== system NDI_and_CA_Model/3Copter_4_NDI&CA/Mass Properties ==
  Arms DCMs : Inport
  CG_0 : Inport  Port=2
  m_0 : Inport  Port=3
  m : Inport  Port=4
  m_M : Inport  Port=5
  I_BAC_0 : Inport  Port=6
  Arm Inertia : MATLAB Function  TreatAsAtomicUnit=on
      settings: PermitHierarchicalResolution=ParametersOnly
  Bus Selector : BusSelector  OutputSignals=T_FaFb,T_FaFb2,T_FaFb3
  CG position : Sum
  Divide : Product  Inputs=*/
  Divide1 : Product  Inputs=**
  Divide2 : Product  Inputs=/*
  Divide3 : Product  Inputs=**
  Motors Pos sum : Sum  Inputs=+++
  Total I_BAC : Sum
  I_BAC : Outport
  CG : Outport  Port=2
  wires:
  Arms DCMs/1 -> Bus Selector/1
  Bus Selector/3 -> Arm Inertia/3(T3_FAFb)  "<T_FaFb3>"
  Bus Selector/2 -> Arm Inertia/2(T2_FAFb)  "<T_FaFb2>"
  Bus Selector/1 -> Arm Inertia/1(T1_FAFb)  "<T_FaFb>"
  Total I_BAC/1 -> I_BAC/1
  m_0/1 -> Divide/1
  m/1 -> Divide/2, Divide2/1
  CG_0/1 -> Divide1/1
  Divide/1 -> Divide1/2
  m_M/1 -> Divide2/2
  CG position/1 -> CG/1
  Divide1/1 -> CG position/1
  Motors Pos sum/1 -> Divide3/1
  Divide2/1 -> Divide3/2
  Divide3/1 -> CG position/2
  Arm Inertia/3(r2_M) -> Motors Pos sum/2
  Arm Inertia/4(r3_M) -> Motors Pos sum/1
  Arm Inertia/1(I_M) -> Total I_BAC/2
  I_BAC_0/1 -> Total I_BAC/1
  Arm Inertia/2(r1_M) -> Motors Pos sum/3

== system NDI_and_CA_Model/3Copter_4_NDI&CA/Normalize Quaternion ==
  q : Inport
  Demux : Demux
  Math Function : Math  Operator=reciprocal  SaturateOnIntegerOverflow=on
  Mux : Mux
  Product{,1..3} (4 alike) : Product  Inputs=**
  Quaternion Modulus : aerolibutil/Quaternion Modulus
  normal(q) : Outport
  wires:
  Product3/1 -> Mux/4
  Product2/1 -> Mux/3
  Product1/1 -> Mux/2
  Product/1 -> Mux/1
  Quaternion Modulus/1 -> Math Function/1
  q/1 -> Demux/1, Quaternion Modulus/1
  Mux/1 -> normal(q)/1
  Demux/1 -> Product/1
  Demux/2 -> Product1/1
  Demux/3 -> Product2/1
  Demux/4 -> Product3/1
  Math Function/1 -> Product3/2, Product2/2, Product/2, Product1/2

== system NDI_and_CA_Model/3Copter_4_SIMPL/6dof Eqs of motion ==
  Forces : Inport
  Moments : Inport  Port=2
  mass : Inport  Port=3
  I_BAC : Inport  Port=4
  CG : Inport  Port=5
  Vb : Inport  Port=6
  q : Inport  Port=7
  omega_b : Inport  Port=8
  Rotational Eq : XXCopter_C/Rotational Eq
  SV_F_b_to_SV_FI : MATLAB Function  TreatAsAtomicUnit=on
      settings: PermitHierarchicalResolution=ParametersOnly
  Translational_Eq : XXCopter_C/Translational_Eq
  q_dot : Subsystem  TreatAsAtomicUnit=on
  Ve : Outport
  Ab : Outport  Port=2
  "q_dot " : Outport  Port=3
  omega_b_dot : Outport  Port=4
  wires:
  I_BAC/1 -> Rotational Eq/3
  mass/1 -> Translational_Eq/5
  Forces/1 -> Translational_Eq/4
  omega_b/1 -> Translational_Eq/2, Rotational Eq/1, q_dot/1(omega_b)
  Rotational Eq/1 -> Translational_Eq/3, omega_b_dot/1
  Translational_Eq/1 -> Ab/1  "A_b"
  CG/1 -> Translational_Eq/6
  q_dot/1(q_dot) -> "q_dot "/1
  SV_F_b_to_SV_FI/1(V_e) -> Ve/1
  Moments/1 -> Rotational Eq/2
  Vb/1 -> Translational_Eq/1, SV_F_b_to_SV_FI/2(V_b)
  q/1 -> SV_F_b_to_SV_FI/1(q), q_dot/2(q)

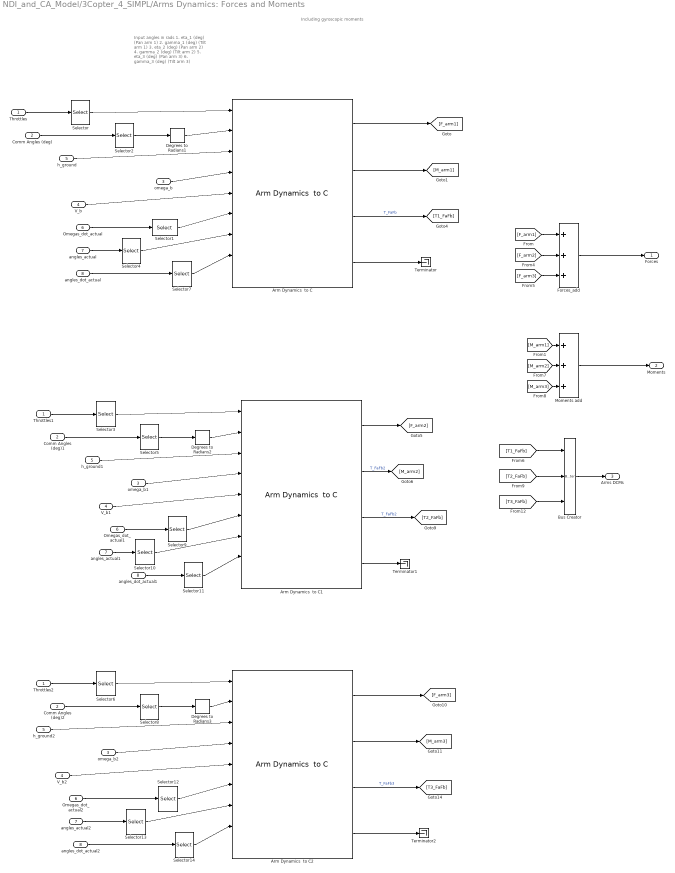
== system NDI_and_CA_Model/3Copter_4_SIMPL/Arms Dynamics: Forces and Moments ==
  note: Including gyroscopic moments
  note: Input angles in rads
      |
      | 1. eta_1 (deg)  (Pan arm 1)
      | 2. gamma_1 (deg)  (Tilt arm 1)
      |
      | 3. eta_2 (deg)  (Pan arm 2)
      | 4. gamma_2 (deg)  (Tilt arm 2)
      |
      | 5. eta_3 (deg)  (Pan arm  3)
      | 6. gamma_3 (deg)  (Tilt arm 3)
  Throttles : Inport
  Comm Angles (deg) : Inport  Port=2
  omega_b : Inport  Port=3
  V_b : Inport  Port=4
  h_ground : Inport  Port=5
  Omegas_dot_actual : Inport  Port=6
  angles_actual : Inport  Port=7
  angles_dot_actual : Inport  Port=8
  Arm Dynamics  to C : XXCopter_C/Arm Dynamics  to C  Rot_sign=Rotation_sign(1)  arm_hub_pos=l*[1;0;0]  Arm_axis=[l_arm;0;0]  arm_num=1  eta_dir=[1;0;0]  gamma_dir=[0;1;0]  J_T=J_T  J_FA=J_FA  h=h  switch_val=direct_feedforward  omega_n=35  xi=1.45  eta_inf_lim=deg2rad(-180)  eta_sup_lim=deg2rad(180)  gamma_inf_lim=deg2rad(-90)  gamma_sup_lim=deg2rad(30)
      link override ESC+Motor Dynamcis  to C/2-D Torque-Throttle-Omega Map: BreakpointsForDimension1=Torque_TTO_vec  BreakpointsForDimension2=Throtle_TTO_vec
  Arm Dynamics  to C1 : XXCopter_C/Arm Dynamics  to C  Rot_sign=Rotation_sign(2)  arm_hub_pos=l*[-1/2;sqrt(3)/2;0]  Arm_axis=[0;l_arm;0]  arm_num=2  eta_dir=[0;1;0]  gamma_dir=[1;0;0]  J_T=J_T  J_FA=J_FA  h=h  switch_val=direct_feedforward  omega_n=35  xi=1.45  eta_inf_lim=deg2rad(-180)  eta_sup_lim=deg2rad(180)  gamma_inf_lim=deg2rad(-30)  gamma_sup_lim=deg2rad(90)
  Arm Dynamics  to C2 : XXCopter_C/Arm Dynamics  to C  Rot_sign=Rotation_sign(3)  arm_hub_pos=l*[-1/2;-sqrt(3)/2;0]  Arm_axis=[0;-l_arm;0]  arm_num=3  eta_dir=[0;1;0]  gamma_dir=[1;0;0]  J_T=J_T  J_FA=J_FA  h=h  switch_val=direct_feedforward  omega_n=35  xi=1.45  eta_inf_lim=deg2rad(-180)  eta_sup_lim=deg2rad(180)  gamma_inf_lim=deg2rad(-90)  gamma_sup_lim=deg2rad(30)
  Bus Creator : BusCreator  Inputs=3
  Comm Angles (deg)1 : InportShadow  Port=2
  Comm Angles (deg)2 : InportShadow  Port=2
  Degrees to Radians1 : simulink_extras/Transformations/Degrees to Radians
  Degrees to Radians2 : simulink_extras/Transformations/Degrees to Radians
  Degrees to Radians3 : simulink_extras/Transformations/Degrees to Radians
  Forces_add : Sum  Inputs=+++
  Moments add : Sum  Inputs=+++
  Omegas_dot_actual1 : InportShadow  Port=6
  Omegas_dot_actual2 : InportShadow  Port=6
  Selector : Selector  IndexMode=Zero-based  InputPortWidth=3  Indices=0
  Selector1 : Selector  IndexMode=Zero-based  InputPortWidth=3  Indices=0
  Selector10 : Selector  IndexMode=Zero-based  InputPortWidth=6  Indices=[2,3]
  Selector11 : Selector  IndexMode=Zero-based  InputPortWidth=6  Indices=[2,3]
  Selector12 : Selector  IndexMode=Zero-based  InputPortWidth=3  Indices=2
  Selector13 : Selector  IndexMode=Zero-based  InputPortWidth=6  Indices=[4,5]
  Selector14 : Selector  IndexMode=Zero-based  InputPortWidth=6  Indices=[4,5]
  Selector2 : Selector  IndexMode=Zero-based  InputPortWidth=6  Indices=[0,1]
  Selector3 : Selector  IndexMode=Zero-based  InputPortWidth=3
  Selector4 : Selector  IndexMode=Zero-based  InputPortWidth=6  Indices=[0,1]
  Selector5 : Selector  IndexMode=Zero-based  InputPortWidth=6  Indices=[2,3]
  Selector6 : Selector  IndexMode=Zero-based  InputPortWidth=3  Indices=2
  Selector7 : Selector  IndexMode=Zero-based  InputPortWidth=6  Indices=[0,1]
  Selector8 : Selector  IndexMode=Zero-based  InputPortWidth=6  Indices=[4,5]
  Selector9 : Selector  IndexMode=Zero-based  InputPortWidth=3
  Terminator : Terminator
  Terminator1 : Terminator
  Terminator2 : Terminator
  Throttles1 : InportShadow
  Throttles2 : InportShadow
  V_b1 : InportShadow  Port=4
  V_b2 : InportShadow  Port=4
  angles_actual1 : InportShadow  Port=7
  angles_actual2 : InportShadow  Port=7
  angles_dot_actual1 : InportShadow  Port=8
  angles_dot_actual2 : InportShadow  Port=8
  h_ground1 : InportShadow  Port=5
  h_ground2 : InportShadow  Port=5
  omega_b1 : InportShadow  Port=3
  omega_b2 : InportShadow  Port=3
  Forces : Outport
  Moments : Outport  Port=2
  Arms DCMs : Outport  Port=3
  wires:
  Throttles/1 -> Selector/1
  Selector/1 -> Arm Dynamics  to C/1
  V_b/1 -> Arm Dynamics  to C/5
  Forces_add/1 -> Forces/1
  Moments add/1 -> Moments/1
  h_ground/1 -> Arm Dynamics  to C/3
  Arm Dynamics  to C/1 -> [F_arm1]
  Arm Dynamics  to C/2 -> [M_arm1]
  [F_arm1] -> Forces_add/1
  [M_arm1] -> Moments add/1
  omega_b/1 -> Arm Dynamics  to C/4
  [F_arm2] -> Forces_add/2
  [F_arm3] -> Forces_add/3
  [M_arm3] -> Moments add/3
  [M_arm2] -> Moments add/2
  Degrees to Radians1/1 -> Arm Dynamics  to C/2
  Comm Angles (deg)/1 -> Selector2/1
  Selector2/1 -> Degrees to Radians1/1
  Arm Dynamics  to C/3 -> [T1_FaFb]  "T_FaFb"
  Throttles1/1 -> Selector3/1
  Selector3/1 -> Arm Dynamics  to C1/1
  V_b1/1 -> Arm Dynamics  to C1/5
  h_ground1/1 -> Arm Dynamics  to C1/3
  omega_b1/1 -> Arm Dynamics  to C1/4
  Degrees to Radians2/1 -> Arm Dynamics  to C1/2
  Comm Angles (deg)1/1 -> Selector5/1
  Selector5/1 -> Degrees to Radians2/1
  Arm Dynamics  to C1/3 -> [T2_FaFb]  "T_FaFb2"
  Throttles2/1 -> Selector6/1
  Selector6/1 -> Arm Dynamics  to C2/1
  V_b2/1 -> Arm Dynamics  to C2/5
  h_ground2/1 -> Arm Dynamics  to C2/3
  Arm Dynamics  to C2/1 -> [F_arm3]
  Arm Dynamics  to C2/2 -> [M_arm3]
  omega_b2/1 -> Arm Dynamics  to C2/4
  Degrees to Radians3/1 -> Arm Dynamics  to C2/2
  Comm Angles (deg)2/1 -> Selector8/1
  Selector8/1 -> Degrees to Radians3/1
  Arm Dynamics  to C2/3 -> [T3_FaFb]  "T_FaFb3"
  Arm Dynamics  to C/4 -> Terminator/1
  Arm Dynamics  to C1/4 -> Terminator1/1
  Arm Dynamics  to C2/4 -> Terminator2/1
  Arm Dynamics  to C1/1 -> [F_arm2]
  Arm Dynamics  to C1/2 -> [M_arm2]  "T_FaFb2"
  Bus Creator/1 -> Arms DCMs/1
  [T1_FaFb] -> Bus Creator/1
  [T2_FaFb] -> Bus Creator/2
  [T3_FaFb] -> Bus Creator/3
  Omegas_dot_actual/1 -> Selector1/1
  Selector1/1 -> Arm Dynamics  to C/6
  angles_actual/1 -> Selector4/1
  Selector4/1 -> Arm Dynamics  to C/7
  angles_dot_actual/1 -> Selector7/1
  Selector7/1 -> Arm Dynamics  to C/8
  Omegas_dot_actual1/1 -> Selector9/1
  Selector9/1 -> Arm Dynamics  to C1/6
  Selector10/1 -> Arm Dynamics  to C1/7
  angles_dot_actual1/1 -> Selector11/1
  angles_actual1/1 -> Selector10/1
  Selector11/1 -> Arm Dynamics  to C1/8
  Omegas_dot_actual2/1 -> Selector12/1
  Selector12/1 -> Arm Dynamics  to C2/6
  Selector13/1 -> Arm Dynamics  to C2/7
  angles_dot_actual2/1 -> Selector14/1
  angles_actual2/1 -> Selector13/1
  Selector14/1 -> Arm Dynamics  to C2/8

== system NDI_and_CA_Model/3Copter_4_SIMPL/Mass Properties ==
  Arms DCMs : Inport
  CG_0 : Inport  Port=2
  m_0 : Inport  Port=3
  m : Inport  Port=4
  m_M : Inport  Port=5
  I_BAC_0 : Inport  Port=6
  Arm Inertia : MATLAB Function  TreatAsAtomicUnit=on
      settings: PermitHierarchicalResolution=ParametersOnly
  Bus Selector : BusSelector  OutputSignals=T_FaFb,T_FaFb2,T_FaFb3
  CG position : Sum
  Divide : Product  Inputs=*/
  Divide1 : Product  Inputs=**
  Divide2 : Product  Inputs=/*
  Divide3 : Product  Inputs=**
  Motors Pos sum : Sum  Inputs=+++
  Total I_BAC : Sum
  I_BAC : Outport
  CG : Outport  Port=2
  wires:
  Arms DCMs/1 -> Bus Selector/1
  Bus Selector/3 -> Arm Inertia/3(T3_FAFb)  "<T_FaFb3>"
  Bus Selector/2 -> Arm Inertia/2(T2_FAFb)  "<T_FaFb2>"
  Bus Selector/1 -> Arm Inertia/1(T1_FAFb)  "<T_FaFb>"
  Total I_BAC/1 -> I_BAC/1
  m_0/1 -> Divide/1
  m/1 -> Divide/2, Divide2/1
  CG_0/1 -> Divide1/1
  Divide/1 -> Divide1/2
  m_M/1 -> Divide2/2
  CG position/1 -> CG/1
  Divide1/1 -> CG position/1
  Motors Pos sum/1 -> Divide3/1
  Divide2/1 -> Divide3/2
  Divide3/1 -> CG position/2
  Arm Inertia/3(r2_M) -> Motors Pos sum/2
  Arm Inertia/4(r3_M) -> Motors Pos sum/1
  Arm Inertia/1(I_M) -> Total I_BAC/2
  I_BAC_0/1 -> Total I_BAC/1
  Arm Inertia/2(r1_M) -> Motors Pos sum/3

== system NDI_and_CA_Model/3Copter_4_SIMPL/Normalize Quaternion ==
  q : Inport
  Demux : Demux
  Math Function : Math  Operator=reciprocal  SaturateOnIntegerOverflow=on
  Mux : Mux
  Product{,1..3} (4 alike) : Product  Inputs=**
  Quaternion Modulus : aerolibutil/Quaternion Modulus
  normal(q) : Outport
  wires:
  Product3/1 -> Mux/4
  Product2/1 -> Mux/3
  Product1/1 -> Mux/2
  Product/1 -> Mux/1
  Quaternion Modulus/1 -> Math Function/1
  q/1 -> Demux/1, Quaternion Modulus/1
  Mux/1 -> normal(q)/1
  Demux/1 -> Product/1
  Demux/2 -> Product1/1
  Demux/3 -> Product2/1
  Demux/4 -> Product3/1
  Math Function/1 -> Product3/2, Product2/2, Product/2, Product1/2

== system NDI_and_CA_Model/3Copter_SIMPL&GRAD/6dof Eqs of motion ==
  Forces : Inport
  Moments : Inport  Port=2
  mass : Inport  Port=3
  I_BAC : Inport  Port=4
  CG : Inport  Port=5
  Vb : Inport  Port=6
  omega_b : Inport  Port=7
  Rotational Eq : XXCopter_C/Rotational Eq
  Translational_Eq : XXCopter_C/Translational_Eq
  Ab : Outport
  omega_b_dot : Outport  Port=2
  wires:
  I_BAC/1 -> Rotational Eq/3
  mass/1 -> Translational_Eq/5
  Forces/1 -> Translational_Eq/4
  omega_b/1 -> Translational_Eq/2, Rotational Eq/1
  Rotational Eq/1 -> Translational_Eq/3, omega_b_dot/1
  Translational_Eq/1 -> Ab/1  "A_b"
  CG/1 -> Translational_Eq/6
  Moments/1 -> Rotational Eq/2
  Vb/1 -> Translational_Eq/1
